simulink model "PUBLISHER_POSE"  (R2018a)
settings: Solver=VariableStepAuto  StartTime=0.0  StopTime=10.0  RelTol=1e-3
undefined symbols (not defined in the file or in its folder): Pose
libraries: robotlib x2
settings Model: Creator=root  LastModifiedBy=root

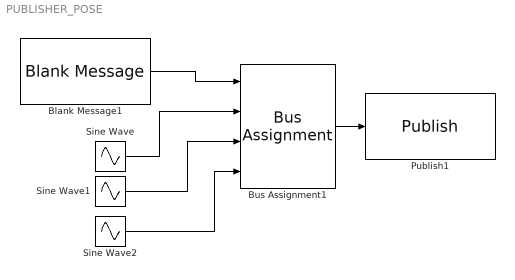
== system PUBLISHER_POSE ==
  Blank Message1 : robotlib/Blank Message  SourceLibraryInfo=This block requires Robotics System Toolbox  messageType=geometry_msgs/PoseStamped  SampleTime=inf
      settings: SourceProductBaseCode=RO
  Bus Assignment1 : BusAssignment  AssignedSignals=Pose.Position.X,Pose.Position.Y,Pose.Position.Z
  Publish1 : robotlib/Publish  SourceLibraryInfo=This block requires Robotics System Toolbox  topicSource=Select from ROS network  topic=/ual/set_pose  messageType=geometry_msgs/PoseStamped  messageQueueLength=1
      settings: SourceProductBaseCode=RO
  Sine Wave : Sin  Amplitude=5  SampleTime=0
  Sine Wave1 : Sin  Frequency=5  SampleTime=0
  Sine Wave2 : Sin  Amplitude=5  Frequency=5  SampleTime=0
  wires:
  Sine Wave/1 -> Bus Assignment1/2
  Blank Message1/1 -> Bus Assignment1/1
  Sine Wave1/1 -> Bus Assignment1/3
  Bus Assignment1/1 -> Publish1/1
  Sine Wave2/1 -> Bus Assignment1/4
